simulink model "total_senario"  (R2019a)
settings: Solver=ode4  StartTime=0.0  StopTime=40  FixedStep=0.001  RelTol=1e-3
libraries: nesl_utility x16, sm_lib x13, simulink x1
(part 3 of 3)

== matlab function total_senario/Desired Joint Trajectory/MATLAB Function13 ==
  data: u input; leftTocenter input; centerToface input; face input; faceTorEar input; qd output; rEar input; rEarTolEar input; lEar input; lEarTolNose input; lNose input; lNoseTorNose input; rNose input; rNoseTocNose input; cNose input; cNoseTorEye input; rEye input; rEyeTolEye input; lEye input; lEyeTocenter input; centerToright input; rightToleft input
function qd = fcn(u, leftTocenter, centerToface, face, faceTorEar,rEar, rEarTolEar,lEar, lEarTolNose,lNose, lNoseTorNose, rNose, rNoseTocNose, cNose, cNoseTorEye, rEye, rEyeTolEye ,lEye, lEyeTocenter, centerToright, rightToleft)
t = u(1);
qd = zeros(4, 1);



if (t < 5)
    qd_buf = leftTocenter;
    qd = [qd_buf(1); qd_buf(2); qd_buf(3); qd_buf(4)];

elseif (t < 6)
    qd_buf = centerToface;
    qd = [qd_buf(1); qd_buf(2); qd_buf(3); qd_buf(4)];

elseif (t < 7)
    qd_buf = face;
    qd = [qd_buf(1); qd_buf(2); qd_buf(3); qd_buf(4)];
    
elseif (t < 8)
    qd_buf = faceTorEar;
    qd = [qd_buf(1); qd_buf(2); qd_buf(3); qd_buf(4)];
    
elseif (t < 9)
    qd_buf = rEar;
    qd = [qd_buf(1); qd_buf(2); qd_buf(3); qd_buf(4)];
    
elseif (t < 10)
    qd_buf = rEarTolEar;
    qd = [qd_buf(1); qd_buf(2); qd_buf(3); qd_buf(4)];
  
elseif (t < 11)
    qd_buf = lEar;
    qd = [qd_buf(1); qd_buf(2); qd_buf(3); qd_buf(4)];

elseif (t < 12)
    qd_buf = lEarTolNose;
    qd = [qd_buf(1); qd_buf(2); qd_buf(3); qd_buf(4)];

elseif (t < 13)
    qd_buf = lNose;
    qd = [qd_buf(1); qd_buf(2); qd_buf(3); qd_buf(4)];
    
elseif (t < 14)
    qd_buf = lNoseTorNose;
    qd = [qd_buf(1); qd_buf(2); qd_buf(3); qd_buf(4)];
    
elseif (t < 15)
    qd_buf = rNose;
    qd = [qd_buf(1); qd_buf(2); qd_buf(3); qd_buf(4)];
    
elseif (t < 16)
    qd_buf = rNoseTocNose;
    qd = [qd_buf(1); qd_buf(2); qd_buf(3); qd_buf(4)];
    
elseif (t < 17)
    qd_buf = cNose;
    qd = [qd_buf(1); qd_buf(2); qd_buf(3); qd_buf(4)];
    
elseif (t < 18)
    qd_buf = cNoseTorEye;
    qd = [qd_buf(1); qd_buf(2); qd_buf(3); qd_buf(4)];
    
elseif (t < 19)
    qd_buf = rEye;
    qd = [qd_buf(1); qd_buf(2); qd_buf(3); qd_buf(4)];
    
elseif (t < 20)
    qd_buf = rEyeTolEye;
    qd = [qd_buf(1); qd_buf(2); qd_buf(3); qd_buf(4)];
        
elseif (t < 21)
    qd_buf = lEye;
    qd = [qd_buf(1); qd_buf(2); qd_buf(3); qd_buf(4)];

elseif (t < 22)
    qd_buf = lEyeTocenter;
    qd = [qd_buf(1); qd_buf(2); qd_buf(3); qd_buf(4)];
    
elseif (t < 27)
    qd_buf = centerToright;
    qd = [qd_buf(1); qd_buf(2); qd_buf(3); qd_buf(4)];  
    
elseif (t <= 37)
    qd_buf = rightToleft;
    qd = [qd_buf(1); qd_buf(2); qd_buf(3); qd_buf(4)];
    
else
    qd = [0; 0; 0; 0];
end


end

== matlab function total_senario/Desired Joint Trajectory/MATLAB Function14 ==
  data: u input; qd output

function qd = fcn(u)
t = u(1);
% time = 0:0.01:10

% (1) r_t,theta_t _ // for Tornado
% cycle=5; % 해당 시간동안 몇바퀴 돌지_진동수
% r_t = 0.1 - (0.1/tf)*t; 
% w_t = cycle*2*pi/tf; 
% theta_t = w_t*t;
% 
% % (2) waffle 중심 cartesian coordinate
% x_wa = r_t.*cos(theta_t); % waffle 중심  
% y_wa = r_t.*sin(theta_t) + 0.4;
% z_wa = - 0.2 - (0.3/tf)*t + 0.6; 
% r_wa = sqrt(x_wa.^2+y_wa.^2);

% psii= atan2(y_wa,x_wa);
% th2 = acos((r_wa.^2+z_wa.^2-L1^2-L2^2)./(2*L1*L2)); % r,z 좌표계로 사이드뷰
% th1 = atan2(z_wa-L3,r_wa) - atan2(L2*sin(th2),L1+L2*cos(th2));
% th3 = pi/2-th1-th2;

x = 0;
y = 0.4;

scale_factor = 1/80;
cycle = 1;
time = 1; %% 20
t=t/time;
w = 2*pi*cycle;
theta = w*t;


psii= psid(t);
th2 = th2d(t); % r,z 좌표계로 사이드뷰
th1 = th1d(t);
th3 = th3d(t);


qd = [psii; th1; th2; th3];

end

function y = s(t)
% if (-1<=t && t<3)
%     y = 2/3*t^3 - 8/27*t^4 +1/27*t^5;
% %     y = 3/2*t^3 - 1*t^4 +3/16*t^5; % 5 / 2
% %     y = 6*t^3 -8*t^4 + 3*t^5; % 5차 1초
% %     y = 2/3*t^2-1/9*t^3; % 3초
% %     y = t^2 - 0.25*t^3; % 2초
% %     y = 2*t^2 - t^3; % 1초
% %     y = t^2;
% elseif (3<=t && t<7)
%     y = t;
% elseif (7<=t &&  t<=10.01)
%     y = -37730/27 + 2600/3*t -5740/27*t^2 + 698/27*t^3 -14/9*t^4 + 1/27*t^5;
% %     y = -10240 + 5825*t -1320*t^2 + 149*t^3 -67/8*t^4 + 3/16*t^5; % 5 / 2
% %     y = -225990 + 119800*t -25380*t^2 + 2686*t^3 -142*t^4 + 3*t^5; % 5차1s
% %     y = 490/9 - 20*t + 8/3*t^2 - 1/9*t^3; % 3초
% %     y = 160 - 55*t +6.5 * t^2 - 0.25*t^3; % 2초
% %     y = 810 - 260*t + 28*t^2 - t^3; % 1초
% %     y = 10 - (t-10)^2;
% else
%     y=t;
% end
y = t;
end


function q = psid(t)

% global L1 L2 L3;
% q = 1.32;
q = atan2(yd(t),xd(t));
% q = 1.32;
end

function q = th1d(t)
L0=1.5;L1=0.3;L2=0.3;L3=0.08; % L3 항상 지면에 수직. 
tf=10; w = 10*pi/tf;
% global L1 L2 L3;
% q = -pi/6;
q = atan2(zd(t)-L3-1.5,sqrt(xd(t)^2+yd(t)^2)) - atan2(L2*sin(th2d(t)),L1+L2*cos(th2d(t)));
% q = -1.52;
end

function q = th2d(t)
L0=1.5;L1=0.3;L2=0.3;L3=0.08; % L3 항상 지면에 수직. 
tf=10; w = 10*pi/tf;
% global L1 L2 L3;
% q = pi/3;
q = acos((xd(t)^2 + yd(t)^2 +(zd(t)-L3-1.5)^2-L1^2-L2^2)/(2*L1*L2));
% q = 1.57;
end

function y = th3d(t)
L0=1.5;L1=0.3;L2=0.3;L3=0.08; % L3 항상 지면에 수직. 
tf=10; w = 10*pi/tf;
% global L1 L2 L3;
y = pi/2 - th1d(t) - th2d(t);
% y = 1.52;
end

function y = xd(t)
L0=1.5;L1=0.3;L2=0.3;L3=0.08; % L3 항상 지면에 수직.
scale_factor = 1/80; cycle = 1;
tf=10; w = 2*pi*cycle;
y =  -0.03125  +0.058962 *cos(0.5*w*t-1.0122)-4.1750e-04- 1.469294361278199e-06;
% global L1 L2 L3 w tf;
% y = ((10 - (10/tf)*(t))*cos(w*(t)))/100;
% y = ((10 - (10/tf)*s(t))*cos(w*s(t)))/100;
% y = (50*cos(pi/4)+(-2*50*cos(pi/4))*s(t)/tf)/100; % 서빙 to 어피치 
end

function y = yd(t)
L0=1.5;L1=0.3;L2=0.3;L3=0.08; % L3 항상 지면에 수직. 
scale_factor = 1/80; cycle = 1;
tf=10; w = 2*pi*cycle;
y = 0.425 +0.058962 *sin(0.5*w*t-1.0122)-1.0582e-04+ 0.00000326818465700;
% global L1 L2 L3 w tf;
% y = ((10 - (10/tf)*(t))*sin(w*(t)) + 40)/100;  % (0,40) 에서 sprial sink./*
% y = ((10 - (10/tf)*s(t))*sin(w*s(t)) + 40)/100;  % (0,40) 에서 sprial sink.
% y = (0.7 .* s(t).*(s(t)-10) + 50*sin(pi/4))/100; % 두배가량 내려감
end

function y = zd(t)
L0=1.5;L1=0.3;L2=0.3;L3=0.08; % L3 항상 지면에 수직. 
scale_factor = 1/80; cycle = 1;
tf=10; w = 2*pi*cycle;
y = 1.3+ 0.000013186867988;
end

== matlab function total_senario/Desired Joint Trajectory/MATLAB Function15 ==
  data: u input; qd output

function qd = fcn(u)
t = u(1);
% time = 0:0.01:10

% (1) r_t,theta_t _ // for Tornado
% cycle=5; % 해당 시간동안 몇바퀴 돌지_진동수
% r_t = 0.1 - (0.1/tf)*t; 
% w_t = cycle*2*pi/tf; 
% theta_t = w_t*t;
% 
% % (2) waffle 중심 cartesian coordinate
% x_wa = r_t.*cos(theta_t); % waffle 중심  
% y_wa = r_t.*sin(theta_t) + 0.4;
% z_wa = - 0.2 - (0.3/tf)*t + 0.6; 
% r_wa = sqrt(x_wa.^2+y_wa.^2);

% psii= atan2(y_wa,x_wa);
% th2 = acos((r_wa.^2+z_wa.^2-L1^2-L2^2)./(2*L1*L2)); % r,z 좌표계로 사이드뷰
% th1 = atan2(z_wa-L3,r_wa) - atan2(L2*sin(th2),L1+L2*cos(th2));
% th3 = pi/2-th1-th2;

x = 0;
y = 0.4;

scale_factor = 1/80;
cycle = 1;
time = 1; %% 20
t=t/time;
w = 2*pi*cycle;
theta = w*t;


psii= psid(t);
th2 = th2d(t); % r,z 좌표계로 사이드뷰
th1 = th1d(t);
th3 = th3d(t);


qd = [psii; th1; th2; th3];

end

function y = s(t)
% if (-1<=t && t<3)
%     y = 2/3*t^3 - 8/27*t^4 +1/27*t^5;
% %     y = 3/2*t^3 - 1*t^4 +3/16*t^5; % 5 / 2
% %     y = 6*t^3 -8*t^4 + 3*t^5; % 5차 1초
% %     y = 2/3*t^2-1/9*t^3; % 3초
% %     y = t^2 - 0.25*t^3; % 2초
% %     y = 2*t^2 - t^3; % 1초
% %     y = t^2;
% elseif (3<=t && t<7)
%     y = t;
% elseif (7<=t &&  t<=10.01)
%     y = -37730/27 + 2600/3*t -5740/27*t^2 + 698/27*t^3 -14/9*t^4 + 1/27*t^5;
% %     y = -10240 + 5825*t -1320*t^2 + 149*t^3 -67/8*t^4 + 3/16*t^5; % 5 / 2
% %     y = -225990 + 119800*t -25380*t^2 + 2686*t^3 -142*t^4 + 3*t^5; % 5차1s
% %     y = 490/9 - 20*t + 8/3*t^2 - 1/9*t^3; % 3초
% %     y = 160 - 55*t +6.5 * t^2 - 0.25*t^3; % 2초
% %     y = 810 - 260*t + 28*t^2 - t^3; % 1초
% %     y = 10 - (t-10)^2;
% else
%     y=t;
% end
y = t;
end


function q = psid(t)

% global L1 L2 L3;
% q = 1.32;
q = atan2(yd(t),xd(t));
% q = 1.32;
end

function q = th1d(t)
L0=1.5;L1=0.3;L2=0.3;L3=0.08; % L3 항상 지면에 수직. 
tf=10; w = 10*pi/tf;
% global L1 L2 L3;
% q = -pi/6;
q = atan2(zd(t)-L3-1.5,sqrt(xd(t)^2+yd(t)^2)) - atan2(L2*sin(th2d(t)),L1+L2*cos(th2d(t)));
% q = -1.52;
end

function q = th2d(t)
L0=1.5;L1=0.3;L2=0.3;L3=0.08; % L3 항상 지면에 수직. 
tf=10; w = 10*pi/tf;
% global L1 L2 L3;
% q = pi/3;
q = acos((xd(t)^2 + yd(t)^2 +(zd(t)-L3-1.5)^2-L1^2-L2^2)/(2*L1*L2));
% q = 1.57;
end

function y = th3d(t)
L0=1.5;L1=0.3;L2=0.3;L3=0.08; % L3 항상 지면에 수직. 
tf=10; w = 10*pi/tf;
% global L1 L2 L3;
y = pi/2 - th1d(t) - th2d(t);
% y = 1.52;
end

function y = xd(t)
L0=1.5;L1=0.3;L2=0.3;L3=0.08; % L3 항상 지면에 수직.
scale_factor = 1/80; cycle = 1;
tf=10; w = 2*pi*cycle;
y =  0.0125 +0.0125*cos(0.5*w*t)-4.1750e-04- 1.469294361278199e-06;
% global L1 L2 L3 w tf;
% y = ((10 - (10/tf)*(t))*cos(w*(t)))/100;
% y = ((10 - (10/tf)*s(t))*cos(w*s(t)))/100;
% y = (50*cos(pi/4)+(-2*50*cos(pi/4))*s(t)/tf)/100; % 서빙 to 어피치 
end

function y = yd(t)
L0=1.5;L1=0.3;L2=0.3;L3=0.08; % L3 항상 지면에 수직. 
scale_factor = 1/80; cycle = 1;
tf=10; w = 2*pi*cycle;
y = 0.375+0.0125 *sin(0.5*w*t)-1.0582e-04+ 0.00000326818465700;
% global L1 L2 L3 w tf;
% y = ((10 - (10/tf)*(t))*sin(w*(t)) + 40)/100;  % (0,40) 에서 sprial sink./*
% y = ((10 - (10/tf)*s(t))*sin(w*s(t)) + 40)/100;  % (0,40) 에서 sprial sink.
% y = (0.7 .* s(t).*(s(t)-10) + 50*sin(pi/4))/100; % 두배가량 내려감
end

function y = zd(t)
L0=1.5;L1=0.3;L2=0.3;L3=0.08; % L3 항상 지면에 수직. 
scale_factor = 1/80; cycle = 1;
tf=10; w = 2*pi*cycle;
y = 1.3+ 0.000013186867988;
end

== matlab function total_senario/Desired Joint Trajectory/MATLAB Function16 ==
  data: u input; qd output

function qd = fcn(u)
t = u(1);
% time = 0:0.01:10

% (1) r_t,theta_t _ // for Tornado
% cycle=5; % 해당 시간동안 몇바퀴 돌지_진동수
% r_t = 0.1 - (0.1/tf)*t; 
% w_t = cycle*2*pi/tf; 
% theta_t = w_t*t;
% 
% % (2) waffle 중심 cartesian coordinate
% x_wa = r_t.*cos(theta_t); % waffle 중심  
% y_wa = r_t.*sin(theta_t) + 0.4;
% z_wa = - 0.2 - (0.3/tf)*t + 0.6; 
% r_wa = sqrt(x_wa.^2+y_wa.^2);

% psii= atan2(y_wa,x_wa);
% th2 = acos((r_wa.^2+z_wa.^2-L1^2-L2^2)./(2*L1*L2)); % r,z 좌표계로 사이드뷰
% th1 = atan2(z_wa-L3,r_wa) - atan2(L2*sin(th2),L1+L2*cos(th2));
% th3 = pi/2-th1-th2;

x = 0;
y = 0.4;

scale_factor = 1/80;
cycle = 1;
time = 1; %% 20
t=t/time;
w = 2*pi*cycle;
theta = w*t;


psii= psid(t);
th2 = th2d(t); % r,z 좌표계로 사이드뷰
th1 = th1d(t);
th3 = th3d(t);


qd = [psii; th1; th2; th3];

end

function y = s(t)
% if (-1<=t && t<3)
%     y = 2/3*t^3 - 8/27*t^4 +1/27*t^5;
% %     y = 3/2*t^3 - 1*t^4 +3/16*t^5; % 5 / 2
% %     y = 6*t^3 -8*t^4 + 3*t^5; % 5차 1초
% %     y = 2/3*t^2-1/9*t^3; % 3초
% %     y = t^2 - 0.25*t^3; % 2초
% %     y = 2*t^2 - t^3; % 1초
% %     y = t^2;
% elseif (3<=t && t<7)
%     y = t;
% elseif (7<=t &&  t<=10.01)
%     y = -37730/27 + 2600/3*t -5740/27*t^2 + 698/27*t^3 -14/9*t^4 + 1/27*t^5;
% %     y = -10240 + 5825*t -1320*t^2 + 149*t^3 -67/8*t^4 + 3/16*t^5; % 5 / 2
% %     y = -225990 + 119800*t -25380*t^2 + 2686*t^3 -142*t^4 + 3*t^5; % 5차1s
% %     y = 490/9 - 20*t + 8/3*t^2 - 1/9*t^3; % 3초
% %     y = 160 - 55*t +6.5 * t^2 - 0.25*t^3; % 2초
% %     y = 810 - 260*t + 28*t^2 - t^3; % 1초
% %     y = 10 - (t-10)^2;
% else
%     y=t;
% end
y = t;
end


function q = psid(t)

% global L1 L2 L3;
% q = 1.32;
q = atan2(yd(t),xd(t));
% q = 1.32;
end

function q = th1d(t)
L0=1.5;L1=0.3;L2=0.3;L3=0.08; % L3 항상 지면에 수직. 
tf=10; w = 10*pi/tf;
% global L1 L2 L3;
% q = -pi/6;
q = atan2(zd(t)-L3-1.5,sqrt(xd(t)^2+yd(t)^2)) - atan2(L2*sin(th2d(t)),L1+L2*cos(th2d(t)));
% q = -1.52;
end

function q = th2d(t)
L0=1.5;L1=0.3;L2=0.3;L3=0.08; % L3 항상 지면에 수직. 
tf=10; w = 10*pi/tf;
% global L1 L2 L3;
% q = pi/3;
q = acos((xd(t)^2 + yd(t)^2 +(zd(t)-L3-1.5)^2-L1^2-L2^2)/(2*L1*L2));
% q = 1.57;
end

function y = th3d(t)
L0=1.5;L1=0.3;L2=0.3;L3=0.08; % L3 항상 지면에 수직. 
tf=10; w = 10*pi/tf;
% global L1 L2 L3;
y = pi/2 - th1d(t) - th2d(t);
% y = 1.52;
end

function y = xd(t)
L0=1.5;L1=0.3;L2=0.3;L3=0.08; % L3 항상 지면에 수직.
scale_factor = 1/80; cycle = 1;
tf=10; w = 2*pi*cycle;
y = 0.015625 +0.0113 *cos(0.5*w*t+2.55359)-4.1750e-04 -2.7168e-05- 1.469294361278199e-06;
% global L1 L2 L3 w tf;
% y = ((10 - (10/tf)*(t))*cos(w*(t)))/100;
% y = ((10 - (10/tf)*s(t))*cos(w*s(t)))/100;
% y = (50*cos(pi/4)+(-2*50*cos(pi/4))*s(t)/tf)/100; % 서빙 to 어피치 
end

function y = yd(t)
L0=1.5;L1=0.3;L2=0.3;L3=0.08; % L3 항상 지면에 수직. 
scale_factor = 1/80; cycle = 1;
tf=10; w = 2*pi*cycle;
y = 0.38125 +0.0113 *sin(0.5*w*t+2.55359)-1.0582e-04+ 1.8113e-05+ 0.00000326818465700;
% global L1 L2 L3 w tf;
% y = ((10 - (10/tf)*(t))*sin(w*(t)) + 40)/100;  % (0,40) 에서 sprial sink./*
% y = ((10 - (10/tf)*s(t))*sin(w*s(t)) + 40)/100;  % (0,40) 에서 sprial sink.
% y = (0.7 .* s(t).*(s(t)-10) + 50*sin(pi/4))/100; % 두배가량 내려감
end

function y = zd(t)
L0=1.5;L1=0.3;L2=0.3;L3=0.08; % L3 항상 지면에 수직. 
scale_factor = 1/80; cycle = 1;
tf=10; w = 2*pi*cycle;
y = 1.3+ 0.000013186867988;
end

== matlab function total_senario/Desired Joint Trajectory/MATLAB Function17 ==
  data: u input; qd output

function qd = fcn(u)
t = u(1);
% time = 0:0.01:10

% (1) r_t,theta_t _ // for Tornado
% cycle=5; % 해당 시간동안 몇바퀴 돌지_진동수
% r_t = 0.1 - (0.1/tf)*t; 
% w_t = cycle*2*pi/tf; 
% theta_t = w_t*t;
% 
% % (2) waffle 중심 cartesian coordinate
% x_wa = r_t.*cos(theta_t); % waffle 중심  
% y_wa = r_t.*sin(theta_t) + 0.4;
% z_wa = - 0.2 - (0.3/tf)*t + 0.6; 
% r_wa = sqrt(x_wa.^2+y_wa.^2);

% psii= atan2(y_wa,x_wa);
% th2 = acos((r_wa.^2+z_wa.^2-L1^2-L2^2)./(2*L1*L2)); % r,z 좌표계로 사이드뷰
% th1 = atan2(z_wa-L3,r_wa) - atan2(L2*sin(th2),L1+L2*cos(th2));
% th3 = pi/2-th1-th2;

x = 0;
y = 0.4;

scale_factor = 1/80;
cycle = 1;
time = 1; %% 20
t=t/time;
w = 2*pi*cycle;
theta = w*t;


psii= psid(t);
th2 = th2d(t); % r,z 좌표계로 사이드뷰
th1 = th1d(t);
th3 = th3d(t);


qd = [psii; th1; th2; th3];

end

function y = s(t)
% if (-1<=t && t<3)
%     y = 2/3*t^3 - 8/27*t^4 +1/27*t^5;
% %     y = 3/2*t^3 - 1*t^4 +3/16*t^5; % 5 / 2
% %     y = 6*t^3 -8*t^4 + 3*t^5; % 5차 1초
% %     y = 2/3*t^2-1/9*t^3; % 3초
% %     y = t^2 - 0.25*t^3; % 2초
% %     y = 2*t^2 - t^3; % 1초
% %     y = t^2;
% elseif (3<=t && t<7)
%     y = t;
% elseif (7<=t &&  t<=10.01)
%     y = -37730/27 + 2600/3*t -5740/27*t^2 + 698/27*t^3 -14/9*t^4 + 1/27*t^5;
% %     y = -10240 + 5825*t -1320*t^2 + 149*t^3 -67/8*t^4 + 3/16*t^5; % 5 / 2
% %     y = -225990 + 119800*t -25380*t^2 + 2686*t^3 -142*t^4 + 3*t^5; % 5차1s
% %     y = 490/9 - 20*t + 8/3*t^2 - 1/9*t^3; % 3초
% %     y = 160 - 55*t +6.5 * t^2 - 0.25*t^3; % 2초
% %     y = 810 - 260*t + 28*t^2 - t^3; % 1초
% %     y = 10 - (t-10)^2;
% else
%     y=t;
% end
y = t;
end


function q = psid(t)

% global L1 L2 L3;
% q = 1.32;
q = atan2(yd(t),xd(t));
% q = 1.32;
end

function q = th1d(t)
L0=1.5;L1=0.3;L2=0.3;L3=0.08; % L3 항상 지면에 수직. 
tf=10; w = 10*pi/tf;
% global L1 L2 L3;
% q = -pi/6;
q = atan2(zd(t)-L3-1.5,sqrt(xd(t)^2+yd(t)^2)) - atan2(L2*sin(th2d(t)),L1+L2*cos(th2d(t)));
% q = -1.52;
end

function q = th2d(t)
L0=1.5;L1=0.3;L2=0.3;L3=0.08; % L3 항상 지면에 수직. 
tf=10; w = 10*pi/tf;
% global L1 L2 L3;
% q = pi/3;
q = acos((xd(t)^2 + yd(t)^2 +(zd(t)-L3-1.5)^2-L1^2-L2^2)/(2*L1*L2));
% q = 1.57;
end

function y = th3d(t)
L0=1.5;L1=0.3;L2=0.3;L3=0.08; % L3 항상 지면에 수직. 
tf=10; w = 10*pi/tf;
% global L1 L2 L3;
y = pi/2 - th1d(t) - th2d(t);
% y = 1.52;
end

function y = xd(t)
L0=1.5;L1=0.3;L2=0.3;L3=0.08; % L3 항상 지면에 수직.
scale_factor = 1/80; cycle = 1;
tf=10; w = 2*pi*cycle;
y =  0.028125 + 0.0252*cos(0.5*w*t+0.5191)-4.1750e-04 -4.9032e-05- 1.469294361278199e-06;
% global L1 L2 L3 w tf;
% y = ((10 - (10/tf)*(t))*cos(w*(t)))/100;
% y = ((10 - (10/tf)*s(t))*cos(w*s(t)))/100;
% y = (50*cos(pi/4)+(-2*50*cos(pi/4))*s(t)/tf)/100; % 서빙 to 어피치 
end

function y = yd(t)
L0=1.5;L1=0.3;L2=0.3;L3=0.08; % L3 항상 지면에 수직. 
scale_factor = 1/80; cycle = 1;
tf=10; w = 2*pi*cycle;
y =  0.4 +0.0252 *sin(0.5*w*t+0.5191)-1.0582e-04 + 3.7918e-05+ 0.00000326818465700;
% global L1 L2 L3 w tf;
% y = ((10 - (10/tf)*(t))*sin(w*(t)) + 40)/100;  % (0,40) 에서 sprial sink./*
% y = ((10 - (10/tf)*s(t))*sin(w*s(t)) + 40)/100;  % (0,40) 에서 sprial sink.
% y = (0.7 .* s(t).*(s(t)-10) + 50*sin(pi/4))/100; % 두배가량 내려감
end

function y = zd(t)
L0=1.5;L1=0.3;L2=0.3;L3=0.08; % L3 항상 지면에 수직. 
scale_factor = 1/80; cycle = 1;
tf=10; w = 2*pi*cycle;
y = 1.3+ 0.000013186867988;
end

== matlab function total_senario/Desired Joint Trajectory/MATLAB Function18 ==
  data: u input; qd output

function qd = fcn(u)
t = u(1);
% time = 0:0.01:10

% (1) r_t,theta_t _ // for Tornado
% cycle=5; % 해당 시간동안 몇바퀴 돌지_진동수
% r_t = 0.1 - (0.1/tf)*t; 
% w_t = cycle*2*pi/tf; 
% theta_t = w_t*t;
% 
% % (2) waffle 중심 cartesian coordinate
% x_wa = r_t.*cos(theta_t); % waffle 중심  
% y_wa = r_t.*sin(theta_t) + 0.4;
% z_wa = - 0.2 - (0.3/tf)*t + 0.6; 
% r_wa = sqrt(x_wa.^2+y_wa.^2);

% psii= atan2(y_wa,x_wa);
% th2 = acos((r_wa.^2+z_wa.^2-L1^2-L2^2)./(2*L1*L2)); % r,z 좌표계로 사이드뷰
% th1 = atan2(z_wa-L3,r_wa) - atan2(L2*sin(th2),L1+L2*cos(th2));
% th3 = pi/2-th1-th2;

x = 0;
y = 0.4;

scale_factor = 1/80;
cycle = 1;
time = 1; %% 20
t=t/time;
w = 2*pi*cycle;
theta = w*t;


psii= psid(t);
th2 = th2d(t); % r,z 좌표계로 사이드뷰
th1 = th1d(t);
th3 = th3d(t);


qd = [psii; th1; th2; th3];

end

function y = s(t)
% if (-1<=t && t<3)
%     y = 2/3*t^3 - 8/27*t^4 +1/27*t^5;
% %     y = 3/2*t^3 - 1*t^4 +3/16*t^5; % 5 / 2
% %     y = 6*t^3 -8*t^4 + 3*t^5; % 5차 1초
% %     y = 2/3*t^2-1/9*t^3; % 3초
% %     y = t^2 - 0.25*t^3; % 2초
% %     y = 2*t^2 - t^3; % 1초
% %     y = t^2;
% elseif (3<=t && t<7)
%     y = t;
% elseif (7<=t &&  t<=10.01)
%     y = -37730/27 + 2600/3*t -5740/27*t^2 + 698/27*t^3 -14/9*t^4 + 1/27*t^5;
% %     y = -10240 + 5825*t -1320*t^2 + 149*t^3 -67/8*t^4 + 3/16*t^5; % 5 / 2
% %     y = -225990 + 119800*t -25380*t^2 + 2686*t^3 -142*t^4 + 3*t^5; % 5차1s
% %     y = 490/9 - 20*t + 8/3*t^2 - 1/9*t^3; % 3초
% %     y = 160 - 55*t +6.5 * t^2 - 0.25*t^3; % 2초
% %     y = 810 - 260*t + 28*t^2 - t^3; % 1초
% %     y = 10 - (t-10)^2;
% else
%     y=t;
% end
y = t;
end


function q = psid(t)

% global L1 L2 L3;
% q = 1.32;
q = atan2(yd(t),xd(t));
% q = 1.32;
end

function q = th1d(t)
L0=1.5;L1=0.3;L2=0.3;L3=0.08; % L3 항상 지면에 수직. 
tf=10; w = 10*pi/tf;
% global L1 L2 L3;
% q = -pi/6;
q = atan2(zd(t)-L3-1.5,sqrt(xd(t)^2+yd(t)^2)) - atan2(L2*sin(th2d(t)),L1+L2*cos(th2d(t)));
% q = -1.52;
end

function q = th2d(t)
L0=1.5;L1=0.3;L2=0.3;L3=0.08; % L3 항상 지면에 수직. 
tf=10; w = 10*pi/tf;
% global L1 L2 L3;
% q = pi/3;
q = acos((xd(t)^2 + yd(t)^2 +(zd(t)-L3-1.5)^2-L1^2-L2^2)/(2*L1*L2));
% q = 1.57;
end

function y = th3d(t)
L0=1.5;L1=0.3;L2=0.3;L3=0.08; % L3 항상 지면에 수직. 
tf=10; w = 10*pi/tf;
% global L1 L2 L3;
y = pi/2 - th1d(t) - th2d(t);
% y = 1.52;
end

function y = xd(t)
L0=1.5;L1=0.3;L2=0.3;L3=0.08; % L3 항상 지면에 수직.
scale_factor = 1/80; cycle = 1;
tf=10; w = 2*pi*cycle;
y =  0.0125 +0.0375 *cos(0.5*w*t+pi) -4.1750e-04 +4.3728e-05 -8.7456e-05 - 1.469294361278199e-06;
% global L1 L2 L3 w tf;
% y = ((10 - (10/tf)*(t))*cos(w*(t)))/100;
% y = ((10 - (10/tf)*s(t))*cos(w*s(t)))/100;
% y = (50*cos(pi/4)+(-2*50*cos(pi/4))*s(t)/tf)/100; % 서빙 to 어피치 
end

function y = yd(t)
L0=1.5;L1=0.3;L2=0.3;L3=0.08; % L3 항상 지면에 수직. 
scale_factor = 1/80; cycle = 1;
tf=10; w = 2*pi*cycle;
y = 0.4125+0.0375 *sin(0.5*w*t+pi)-1.0582e-04+3.9610e-05+ 0.00000326818465700;
% global L1 L2 L3 w tf;
% y = ((10 - (10/tf)*(t))*sin(w*(t)) + 40)/100;  % (0,40) 에서 sprial sink./*
% y = ((10 - (10/tf)*s(t))*sin(w*s(t)) + 40)/100;  % (0,40) 에서 sprial sink.
% y = (0.7 .* s(t).*(s(t)-10) + 50*sin(pi/4))/100; % 두배가량 내려감
end

function y = zd(t)
L0=1.5;L1=0.3;L2=0.3;L3=0.08; % L3 항상 지면에 수직. 
scale_factor = 1/80; cycle = 1;
tf=10; w = 2*pi*cycle;
y = 1.3+ 0.000013186867988;
end

== matlab function total_senario/Desired Joint Trajectory/MATLAB Function19 ==
  data: u input; qd output

function qd = fcn(u)
t = u(1);
% time = 0:0.01:10

% (1) r_t,theta_t _ // for Tornado
% cycle=5; % 해당 시간동안 몇바퀴 돌지_진동수
% r_t = 0.1 - (0.1/tf)*t; 
% w_t = cycle*2*pi/tf; 
% theta_t = w_t*t;
% 
% % (2) waffle 중심 cartesian coordinate
% x_wa = r_t.*cos(theta_t); % waffle 중심  
% y_wa = r_t.*sin(theta_t) + 0.4;
% z_wa = - 0.2 - (0.3/tf)*t + 0.6; 
% r_wa = sqrt(x_wa.^2+y_wa.^2);

% psii= atan2(y_wa,x_wa);
% th2 = acos((r_wa.^2+z_wa.^2-L1^2-L2^2)./(2*L1*L2)); % r,z 좌표계로 사이드뷰
% th1 = atan2(z_wa-L3,r_wa) - atan2(L2*sin(th2),L1+L2*cos(th2));
% th3 = pi/2-th1-th2;

x = 0;
y = 0.4;

scale_factor = 1/80;
cycle = 1;
time = 1; %% 20
t=t/time;
w = 2*pi*cycle;
theta = w*t;


psii= psid(t);
th2 = th2d(t); % r,z 좌표계로 사이드뷰
th1 = th1d(t);
th3 = th3d(t);


qd = [psii; th1; th2; th3];

end

function y = s(t)
% if (-1<=t && t<3)
%     y = 2/3*t^3 - 8/27*t^4 +1/27*t^5;
% %     y = 3/2*t^3 - 1*t^4 +3/16*t^5; % 5 / 2
% %     y = 6*t^3 -8*t^4 + 3*t^5; % 5차 1초
% %     y = 2/3*t^2-1/9*t^3; % 3초
% %     y = t^2 - 0.25*t^3; % 2초
% %     y = 2*t^2 - t^3; % 1초
% %     y = t^2;
% elseif (3<=t && t<7)
%     y = t;
% elseif (7<=t &&  t<=10.01)
%     y = -37730/27 + 2600/3*t -5740/27*t^2 + 698/27*t^3 -14/9*t^4 + 1/27*t^5;
% %     y = -10240 + 5825*t -1320*t^2 + 149*t^3 -67/8*t^4 + 3/16*t^5; % 5 / 2
% %     y = -225990 + 119800*t -25380*t^2 + 2686*t^3 -142*t^4 + 3*t^5; % 5차1s
% %     y = 490/9 - 20*t + 8/3*t^2 - 1/9*t^3; % 3초
% %     y = 160 - 55*t +6.5 * t^2 - 0.25*t^3; % 2초
% %     y = 810 - 260*t + 28*t^2 - t^3; % 1초
% %     y = 10 - (t-10)^2;
% else
%     y=t;
% end
y = t;
end


function q = psid(t)

% global L1 L2 L3;
% q = 1.32;
q = atan2(yd(t),xd(t));
% q = 1.32;
end

function q = th1d(t)
L0=1.5;L1=0.3;L2=0.3;L3=0.08; % L3 항상 지면에 수직. 
tf=10; w = 10*pi/tf;
% global L1 L2 L3;
% q = -pi/6;
q = atan2(zd(t)-L3-1.5,sqrt(xd(t)^2+yd(t)^2)) - atan2(L2*sin(th2d(t)),L1+L2*cos(th2d(t)));
% q = -1.52;
end

function q = th2d(t)
L0=1.5;L1=0.3;L2=0.3;L3=0.08; % L3 항상 지면에 수직. 
tf=10; w = 10*pi/tf;
% global L1 L2 L3;
% q = pi/3;
q = acos((xd(t)^2 + yd(t)^2 +(zd(t)-L3-1.5)^2-L1^2-L2^2)/(2*L1*L2));
% q = 1.57;
end

function y = th3d(t)
L0=1.5;L1=0.3;L2=0.3;L3=0.08; % L3 항상 지면에 수직. 
tf=10; w = 10*pi/tf;
% global L1 L2 L3;
y = pi/2 - th1d(t) - th2d(t);
% y = 1.52;
end

function y = xd(t)
L0=1.5;L1=0.3;L2=0.3;L3=0.08; % L3 항상 지면에 수직.
scale_factor = 1/80; cycle = 1;
tf=10; w = 2*pi*cycle;
y = 0.05+0.05*cos(0.5*w*t) - 1.469294361278199e-06;
% global L1 L2 L3 w tf;
% y = ((10 - (10/tf)*(t))*cos(w*(t)))/100;
% y = ((10 - (10/tf)*s(t))*cos(w*s(t)))/100;
% y = (50*cos(pi/4)+(-2*50*cos(pi/4))*s(t)/tf)/100; % 서빙 to 어피치 
end

function y = yd(t)
L0=1.5;L1=0.3;L2=0.3;L3=0.08; % L3 항상 지면에 수직. 
scale_factor = 1/80; cycle = 1;
tf=10; w = 2*pi*cycle;
y = 0.4+0.05*sin(0.5*w*t) + 0.00000326818465700;
% global L1 L2 L3 w tf;
% y = ((10 - (10/tf)*(t))*sin(w*(t)) + 40)/100;  % (0,40) 에서 sprial sink./*
% y = ((10 - (10/tf)*s(t))*sin(w*s(t)) + 40)/100;  % (0,40) 에서 sprial sink.
% y = (0.7 .* s(t).*(s(t)-10) + 50*sin(pi/4))/100; % 두배가량 내려감
end

function y = zd(t)
L0=1.5;L1=0.3;L2=0.3;L3=0.08; % L3 항상 지면에 수직. 
scale_factor = 1/80; cycle = 1;
tf=10; w = 2*pi*cycle;
y = 1.3 + 0.000013186867988;
end

== matlab function total_senario/Desired Joint Trajectory/MATLAB Function20 ==
  data: u input; qd output

function qd = fcn(u)
t = u(1);
t = t - 22;

psii= psid(t);
th2 = th2d(t); % r,z 좌표계로 사이드뷰
th1 = th1d(t);
th3 = th3d(t);

qd = [psii; th1; th2; th3];
end


function q = psid(t)


if -1<=t && t<0.9778
    q = 7079457343025333/4503599627370496 - t^2/10;
elseif 0.9778<=t && t<4.0023
    q = 1352881985075210612543874782426921/811296384146066816957890051440640 - (7045467285855423*t)/36028797018963968;
elseif 4.0023<=t && t<=6
    q = (t - 141520394443479/35184372088832)^2/10 - (7045467285855423*t)/36028797018963968 + 1352881985075210612543874782426921/811296384146066816957890051440640;
else
    q=0;
end

end

function q = th1d(t)
if -1<=t && t<0.5716
    q = t^2/10 - 1386130790860819/1125899906842624;
elseif 0.5716<=t && t<4.4284
    q = (4118595902425847*t)/36028797018963968 - 71145653496126529178201387/56294995342131200000000000;
elseif 4.4284<=t && t<=6
    q = (4118595902425847*t)/36028797018963968 - (t - 2492984010666239/562949953421312)^2/10 - 71145653496126529178201387/56294995342131200000000000;
else
    q=0;
end
end

function q = th2d(t)
if -1<=t && t<0.1108
    q = 1396913695184541/1125899906842624 - t^2/10;
elseif 0.1108<=t && t<4.8893
    q = 139829492415024160313660151/112589990684262400000000000 - (6384879292512719*t)/288230376151711744;
elseif 4.8893<=t && t<=6
    q = (t - 2752452164047343/562949953421312)^2/10 - (6384879292512719*t)/288230376151711744 + 139829492415024160313660151/112589990684262400000000000;
else
    q=0;
end
end

function y = th3d(t)
y = pi/2 - th1d(t) - th2d(t);
end

== matlab function total_senario/Desired Joint Trajectory/MATLAB Function21 ==
  data: t input; qd output

function qd = fcn(t)
t = t-27;
% time = 0:0.01:10

% (1) r_t,theta_t _ // for Tornado
% cycle=5; % 해당 시간동안 몇바퀴 돌지_진동수
% r_t = 0.1 - (0.1/tf)*t; 
% w_t = cycle*2*pi/tf; 
% theta_t = w_t*t;
% 
% % (2) waffle 중심 cartesian coordinate
% x_wa = r_t.*cos(theta_t); % waffle 중심  
% y_wa = r_t.*sin(theta_t) + 0.4;
% z_wa = - 0.2 - (0.3/tf)*t + 0.6; 
% r_wa = sqrt(x_wa.^2+y_wa.^2);

% psii= atan2(y_wa,x_wa);
% th2 = acos((r_wa.^2+z_wa.^2-L1^2-L2^2)./(2*L1*L2)); % r,z 좌표계로 사이드뷰
% th1 = atan2(z_wa-L3,r_wa) - atan2(L2*sin(th2),L1+L2*cos(th2));
% th3 = pi/2-th1-th2;

x = 0;
y = 0.4;

scale_factor = 1/80;
cycle = 1;
time = 1; %% 20
t=t/time;
w = 2*pi*cycle;
theta = w*t;

psii= psid(t);
th2 = th2d(t); % r,z 좌표계로 사이드뷰
th1 = th1d(t);
th3 = th3d(t);


% psii= psid(t);
% th2 = th2d(t); % r,z 좌표계로 사이드뷰
% th1 = th1d(t);
% th3 = th3d(t);


qd = [psii; th1; th2; th3];

end

function y = s(t)
% if (-1<=t && t<3)
%     y = 2/3*t^3 - 8/27*t^4 +1/27*t^5;
% %     y = 3/2*t^3 - 1*t^4 +3/16*t^5; % 5 / 2
% %     y = 6*t^3 -8*t^4 + 3*t^5; % 5차 1초
% %     y = 2/3*t^2-1/9*t^3; % 3초
% %     y = t^2 - 0.25*t^3; % 2초
% %     y = 2*t^2 - t^3; % 1초
% %     y = t^2;
% elseif (3<=t && t<7)
%     y = t;
% elseif (7<=t &&  t<=10.01)
%     y = -37730/27 + 2600/3*t -5740/27*t^2 + 698/27*t^3 -14/9*t^4 + 1/27*t^5;
% %     y = -10240 + 5825*t -1320*t^2 + 149*t^3 -67/8*t^4 + 3/16*t^5; % 5 / 2
% %     y = -225990 + 119800*t -25380*t^2 + 2686*t^3 -142*t^4 + 3*t^5; % 5차1s
% %     y = 490/9 - 20*t + 8/3*t^2 - 1/9*t^3; % 3초
% %     y = 160 - 55*t +6.5 * t^2 - 0.25*t^3; % 2초
% %     y = 810 - 260*t + 28*t^2 - t^3; % 1초
% %     y = 10 - (t-10)^2;
% else
%     y=t;
% end
y = t;
end

function q = psid(t)

% global L1 L2 L3;
% q = 1.32;
q = atan2(yd(t),xd(t));
% q = 1.32;
end

function q = th1d(t)
L0=1.5;L1=0.3;L2=0.3;L3=0.08; % L3 항상 지면에 수직. 
tf=10; w = 10*pi/tf;
% global L1 L2 L3;
% q = -pi/6;
q = atan2(zd(t)-L3-1.5,sqrt(xd(t)^2+yd(t)^2)) - atan2(L2*sin(th2d(t)),L1+L2*cos(th2d(t)));
% q = -1.52;
end

function q = th2d(t)
L0=1.5;L1=0.3;L2=0.3;L3=0.08; % L3 항상 지면에 수직. 
tf=10; w = 10*pi/tf;
% global L1 L2 L3;
% q = pi/3;
q = acos((xd(t)^2 + yd(t)^2 +(zd(t)-L3-1.5)^2-L1^2-L2^2)/(2*L1*L2));
% q = 1.57;
end

function y = th3d(t)
L0=1.5;L1=0.3;L2=0.3;L3=0.08; % L3 항상 지면에 수직. 
tf=10; w = 10*pi/tf;
% global L1 L2 L3;
y = pi/2 - th1d(t) - th2d(t);
% y = 1.52;
end

function y = xd(t)
L0=1.5;L1=0.3;L2=0.3;L3=0.08; % L3 항상 지면에 수직.
scale_factor = 1/80; cycle = 1;
tf=10; w = 2*pi*cycle;
y = (50*cos(pi/4)+(-2*50*cos(pi/4))*s(t)/tf)/100 + 2.223734486717088e-06; % 4번
end

function y = yd(t)
L0=1.5;L1=0.3;L2=0.3;L3=0.08; % L3 항상 지면에 수직. 
scale_factor = 1/80; cycle = 1;
tf=10; w = 2*pi*cycle;
y = (0.7 .* s(t).*(s(t)-10) + 50*sin(pi/4))/100 + 3.522422173218853e-06; % 4번
% global L1 L2 L3 w tf;
% y = ((10 - (10/tf)*(t))*sin(w*(t)) + 40)/100;  % (0,40) 에서 sprial sink./*
% y = ((10 - (10/tf)*s(t))*sin(w*s(t)) + 40)/100;  % (0,40) 에서 sprial sink.
% y = (0.7 .* s(t).*(s(t)-10) + 50*sin(pi/4))/100; % 두배가량 내려감
end

function y = zd(t)
L0=1.5;L1=0.3;L2=0.3;L3=0.08; % L3 항상 지면에 수직. 
scale_factor = 1/80; cycle = 1;
tf=10; w = 2*pi*cycle;
y = (150 -0.8.*s(t).*(s(t)-10))/100 -2.359176267896501e-05 ; % 4번
end

== matlab function total_senario/Desired Joint Trajectory/MATLAB Function22 ==
  data: u input; y output
function y = fcn(u)
t = u(1);
if t<27
    y = 27;
elseif (t<=37)
    y = t;
else
    y=10;
end
 
    
end

== matlab function total_senario/Desired Joint Trajectory/MATLAB Function23 ==
  data: u input; qd output

function qd = fcn(u)
t = u(1);
% time = 0:0.01:10

% (1) r_t,theta_t _ // for Tornado
% cycle=5; % 해당 시간동안 몇바퀴 돌지_진동수
% r_t = 0.1 - (0.1/tf)*t; 
% w_t = cycle*2*pi/tf; 
% theta_t = w_t*t;
% 
% % (2) waffle 중심 cartesian coordinate
% x_wa = r_t.*cos(theta_t); % waffle 중심  
% y_wa = r_t.*sin(theta_t) + 0.4;
% z_wa = - 0.2 - (0.3/tf)*t + 0.6; 
% r_wa = sqrt(x_wa.^2+y_wa.^2);

% psii= atan2(y_wa,x_wa);
% th2 = acos((r_wa.^2+z_wa.^2-L1^2-L2^2)./(2*L1*L2)); % r,z 좌표계로 사이드뷰
% th1 = atan2(z_wa-L3,r_wa) - atan2(L2*sin(th2),L1+L2*cos(th2));
% th3 = pi/2-th1-th2;

x = 0;
y = 0.4;

scale_factor = 1/80;
cycle = 1;
time = 1; %% 20
t=t/time;
w = 2*pi*cycle;
theta = w*t;


psii= psid(t);
th2 = th2d(t); % r,z 좌표계로 사이드뷰
th1 = th1d(t);
th3 = th3d(t);


qd = [psii; th1; th2; th3];

end

function y = s(t)
% if (-1<=t && t<3)
%     y = 2/3*t^3 - 8/27*t^4 +1/27*t^5;
% %     y = 3/2*t^3 - 1*t^4 +3/16*t^5; % 5 / 2
% %     y = 6*t^3 -8*t^4 + 3*t^5; % 5차 1초
% %     y = 2/3*t^2-1/9*t^3; % 3초
% %     y = t^2 - 0.25*t^3; % 2초
% %     y = 2*t^2 - t^3; % 1초
% %     y = t^2;
% elseif (3<=t && t<7)
%     y = t;
% elseif (7<=t &&  t<=10.01)
%     y = -37730/27 + 2600/3*t -5740/27*t^2 + 698/27*t^3 -14/9*t^4 + 1/27*t^5;
% %     y = -10240 + 5825*t -1320*t^2 + 149*t^3 -67/8*t^4 + 3/16*t^5; % 5 / 2
% %     y = -225990 + 119800*t -25380*t^2 + 2686*t^3 -142*t^4 + 3*t^5; % 5차1s
% %     y = 490/9 - 20*t + 8/3*t^2 - 1/9*t^3; % 3초
% %     y = 160 - 55*t +6.5 * t^2 - 0.25*t^3; % 2초
% %     y = 810 - 260*t + 28*t^2 - t^3; % 1초
% %     y = 10 - (t-10)^2;
% else
%     y=t;
% end
y = t;
end


function q = psid(t)

% global L1 L2 L3;
% q = 1.32;
q = atan2(yd(t),xd(t));
% q = 1.32;
end

function q = th1d(t)
L0=1.5;L1=0.3;L2=0.3;L3=0.08; % L3 항상 지면에 수직. 
tf=10; w = 10*pi/tf;
% global L1 L2 L3;
% q = -pi/6;
q = atan2(zd(t)-L3-1.5,sqrt(xd(t)^2+yd(t)^2)) - atan2(L2*sin(th2d(t)),L1+L2*cos(th2d(t)));
% q = -1.52;
end

function q = th2d(t)
L0=1.5;L1=0.3;L2=0.3;L3=0.08; % L3 항상 지면에 수직. 
tf=10; w = 10*pi/tf;
% global L1 L2 L3;
% q = pi/3;
q = acos((xd(t)^2 + yd(t)^2 +(zd(t)-L3-1.5)^2-L1^2-L2^2)/(2*L1*L2));
% q = 1.57;
end

function y = th3d(t)
L0=1.5;L1=0.3;L2=0.3;L3=0.08; % L3 항상 지면에 수직. 
tf=10; w = 10*pi/tf;
% global L1 L2 L3;
y = pi/2 - th1d(t) - th2d(t);
% y = 1.52;
end

function y = xd(t)
L0=1.5;L1=0.3;L2=0.3;L3=0.08; % L3 항상 지면에 수직.
scale_factor = 1/80; cycle = 1;
tf=10; w = 2*pi*cycle;
y = 0.0125+0.075*cos(-0.5*w*t+pi)-4.1750e-04- 1.469294361278199e-06;
% y = 0.0125+0.075*cos(0.5*w*(10-t)-pi);
% y = 0.0125+0.075*cos(-pi/2);
% global L1 L2 L3 w tf;
% y = ((10 - (10/tf)*(t))*cos(w*(t)))/100;
% y = ((10 - (10/tf)*s(t))*cos(w*s(t)))/100;
% y = (50*cos(pi/4)+(-2*50*cos(pi/4))*s(t)/tf)/100; % 서빙 to 어피치 
end

function y = yd(t)
L0=1.5;L1=0.3;L2=0.3;L3=0.08; % L3 항상 지면에 수직. 
scale_factor = 1/80; cycle = 1;
tf=10; w = 2*pi*cycle;
y = 0.475+0.075*sin(-0.5*w*t+pi)-1.0582e-04+ 0.00000326818465700;
% y = 0.475+0.075*sin(0.5*w*(10-t)-pi);
% y = 0.475+0.075*sin(-pi/2);
% global L1 L2 L3 w tf;
% y = ((10 - (10/tf)*(t))*sin(w*(t)) + 40)/100;  % (0,40) 에서 sprial sink./*
% y = ((10 - (10/tf)*s(t))*sin(w*s(t)) + 40)/100;  % (0,40) 에서 sprial sink.
% y = (0.7 .* s(t).*(s(t)-10) + 50*sin(pi/4))/100; % 두배가량 내려감
end

function y = zd(t)
y = 1.3+ 0.000013186867988;
end

== matlab function total_senario/Desired Joint Trajectory/MATLAB Function24 ==
  data: u input; s output
function s = fcn(u)
t = u(1);
n = fix(t/1);
y = 0;
t = t-n;

if n<=4
    y = n + t;
elseif n <= 21
    if 0<=t && t<=0.3
        y = 200/3*t^3 -8000/27*t^4 + 10000/27*t^5 + n; % 0.3
    elseif 0.3<t && t<0.7
        y = t + n;
    elseif 0.7<=t &&  t<1
        y = -3773/27 + 2600/3*t -57400/27*t^2 + 69800/27*t^3 -14000/9*t^4 +10000/27*t^5 + n;% 0.7
    end
elseif n <= 26
    y = n + t;
elseif n <= 36
    if 0<=(t+n-27) && (t+n-27)<=3
        y = 2/3*(t+n-27)^3 - 8/27*(t+n-27)^4 +1/27*(t+n-27)^5 + 27;
    elseif 3<(t+n-27) && (t+n-27)<7
        y = t + n;
    elseif 7<=(t+n-27) &&  (t+n-27)<10
        y = -37730/27 + 2600/3*(t+n-27) -5740/27*(t+n-27)^2 + 698/27*(t+n-27)^3 -14/9*(t+n-27)^4 + 1/27*(t+n-27)^5 +27;
    end
else
    y = 37;
end

s = y;

== matlab function total_senario/MATLAB Function ==
  data: x output; psii input; y output; th1 input; th2 input; th3 input; z output
function [x,y,z] = fcn(psii, th1, th2, th3)

L1 = 0.3;
L2 = 0.3;
L3 = 0.08;

x = (L1*cos(th1) + L2*cos(th1+th2) + L3*cos(th1+th2+th3))*cos(psii);
y = (L1*cos(th1) + L2*cos(th1+th2) + L3*cos(th1+th2+th3))*sin(psii);
z = (L1*sin(th1) + L2*sin(th1+th2) + L3*sin(th1+th2+th3)) + 1.5;
